simulink model "k6jca_181222_SHERA_2_subsample"  (R2018b)
settings: Solver=ode45  StartTime=0.0  StopTime=10000  MaxStep=1  RelTol=1e-3  EnableMultiTasking=on
InitFcn:
  | D=30
settings Model: Creator=Dick  LastModifiedBy=Jeff
settings DataIOCC: LimitDataPoints=on  SaveFormat=Array  SaveOutput=off  SignalLogging=off  DSMLogging=off  SaveTime=off
settings OptimizationCC: LifeSpan=inf
settings DebuggingCC: SFUnexpectedBacktrackingDiag=warning  SFNoUnconditionalDefaultTransitionDiag=warning  SFExecutionAtInitializationDiag=none
settings HardwareCC: ProdBitPerPointer=32  ProdBitPerSizeT=32  ProdBitPerPtrDiffT=32  ProdLargestAtomicFloat=None  ProdIntDivRoundTo=Undefined  ProdEndianess=Unspecified  ProdWordSize=32  ProdHWDeviceType=32-bit Generic
settings ModelReferenceCC: PropagateSignalLabelsOutOfModel=off
settings SFSimCC: SimUseLocalCustomCode=off
settings RTWCC: RTWUseLocalCustomCode=off
settings CodeAppCC: StateflowObjectComments=on
settings GRTTargetCC: TargetLangStandard=C89/C90 (ANSI)  GeneratePreprocessorConditionals=Disable all
settings ConfigComp: CovMetricSettings=dw  CovHtmlReporting=on  CovSaveCumulativeToWorkspaceVar=on  CovSaveSingleToWorkspaceVar=on  CovExternalEMLEnable=off

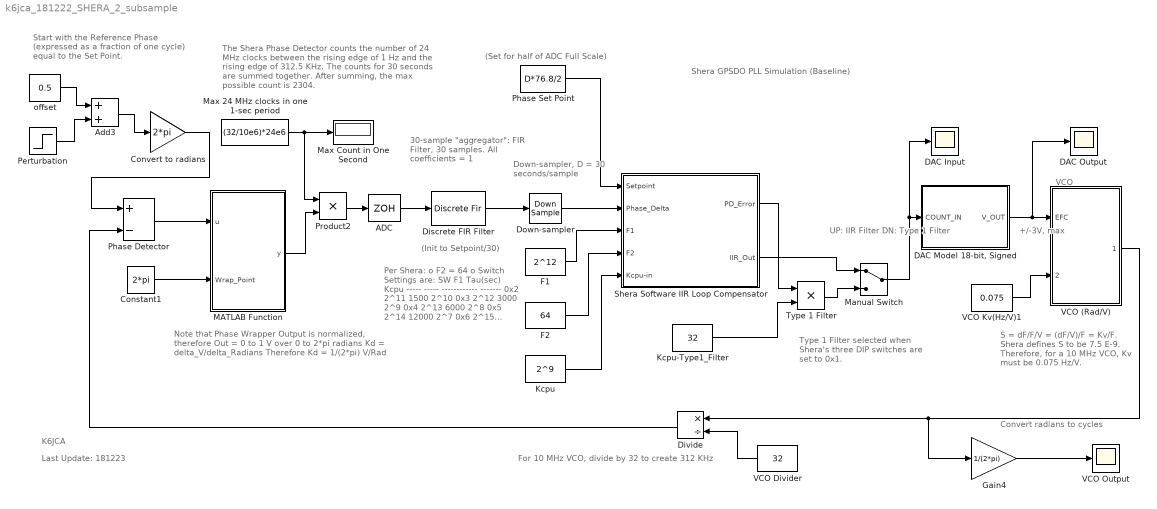
== system k6jca_181222_SHERA_2_subsample ==
  note: Down-sampler,
      | D = 30
      | seconds/sample
  note: Last Update: 181223
  note: (Set for half of ADC Full Scale)
  note: 30-sample "aggregator":
      | FIR Filter,
      | 30 samples.
      | All coefficients = 1
  note: Start with the Reference Phase
      | (expressed as a fraction of one cycle)
      | equal to the Set Point.
  note: UP:  IIR Filter
      | DN:  Type 1 Filter
  note: Type 1 Filter selected
      | when Shera's three
      | DIP switches are set to 0x1.
  note: S = dF/F/V = (dF/V)/F = Kv/F.
      | Shera defines S to be 7.5 E-9.
      | Therefore, for a 10 MHz VCO,
      | Kv must be 0.075 Hz/V.
  note: The Shera Phase Detector counts the number of 24 MHz clocks between the rising edge of 1 Hz and the rising edge of 312.5 KHz.
      |
      | The counts for 30 seconds are summed together.  After summing,  the max possible count is 2304.
  note: Per Shera:
      |      o  F2 = 64
      |      o  Switch Settings are:
      |
      |    SW      F1     Tau(sec)    Kcpu
      |    -----     -----    ------------   -------
      |    0x2     2^11      1500       2^10
      |    0x3     2^12      3000       2^9
      |    0x4     2^13      6000       2^8
      |    0x5     2^14    12000       2^7
      |    0x6     2^15    24000       2^6
      |    0x7     2^16    48000       2^5
  note: For 10 MHz VCO, divide by 32 to create 312 KHz
  note: +/-3V,
      |  max
  note: K6JCA
  note: Shera GPSDO PLL Simulation
      | (Baseline)
  note: Convert radians to cycles
  note: Note that Phase Wrapper Output is normalized,
      | therefore Out =  0 to 1 V over 0 to 2*pi radians
      |
      | Kd = delta_V/delta_Radians
      | Therefore Kd = 1/(2*pi)  V/Rad
  note: VCO
  note: (Init to Setpoint/30)
  ADC : ZeroOrderHold
  Add3 : Sum
  Constant1 : Constant  Value=2*pi  SampleTime=Inf
  "Convert to radians " : Gain  Gain=2*pi
  DAC Input : Scope
  "DAC Model 18-bit, Signed" : Subsystem
  DAC Output : Scope
  Discrete FIR Filter : DiscreteFir  Coefficients=[1 1 1 1 1 1 1 1 1 1 1 1 1 1 1 1 1 1 1 1 1 1 1 1 1 1 1 1 1 1]  InitialStates=76.8/2
  Divide : Product  Inputs=*/
  "Down-sampler " : DownSample  N=D  RateOptions=Allow multirate processing
  F1 : Constant  Value=2^12  SampleTime=Inf
  F2 : Constant  Value=64  SampleTime=Inf
  Gain4 : Gain  Gain=1/(2*pi)
  Kcpu : Constant  Value=2^9  SampleTime=Inf
  Kcpu-Type1_Filter : Constant  Value=32  SampleTime=Inf
  MATLAB Function : MATLAB Function  TreatAsAtomicUnit=on
  Manual Switch : ManualSwitch
  Max 24 MHz clocks in one 1-sec period : Constant  Value=(32/10e6)*24e6  SampleTime=Inf
  Max Count in One Second : Display
  "Perturbation " : Step  Time=100  After=0.49  SampleTime=1
  Phase Detector : Sum  Inputs=+-
  Phase Set Point : Constant  Value=D*76.8/2  SampleTime=Inf
  Product2 : Product
  "Shera Software IIR Loop Compensator " : Subsystem
  Type 1 Filter : Product  Inputs=**
  VCO (Rad/V) : Subsystem
  VCO Divider : Constant  Value=32  SampleTime=Inf
  VCO Kv(Hz/V)1 : Constant  Value=0.075  SampleTime=Inf
  VCO Output : Scope
  offset : Constant  Value=0.5  SampleTime=Inf
  wires:
  "Perturbation "/1 -> Add3/2
  Phase Detector/1 -> MATLAB Function/1(u)
  Constant1/1 -> MATLAB Function/2(Wrap_Point)
  Product2/1 -> ADC/1
  "Convert to radians "/1 -> Phase Detector/1
  "Shera Software IIR Loop Compensator "/1("PD_Error ") -> Type 1 Filter/1
  VCO (Rad/V)/1(Radians) -> Divide/1, Gain4/1
  F2/1 -> "Shera Software IIR Loop Compensator "/4(F2)
  F1/1 -> "Shera Software IIR Loop Compensator "/3(F1)
  Kcpu/1 -> "Shera Software IIR Loop Compensator "/5(Kcpu-in)
  VCO Kv(Hz/V)1/1 -> VCO (Rad/V)/2(Kv_(Hz/V))
  "DAC Model 18-bit, Signed"/1(V_OUT) -> DAC Output/1, VCO (Rad/V)/1(EFC)
  VCO Divider/1 -> Divide/2
  Manual Switch/1 -> DAC Input/1, "DAC Model 18-bit, Signed"/1(COUNT_IN)
  Kcpu-Type1_Filter/1 -> Type 1 Filter/2
  Type 1 Filter/1 -> Manual Switch/2
  "Shera Software IIR Loop Compensator "/2("IIR_Out ") -> Manual Switch/1
  Phase Set Point/1 -> "Shera Software IIR Loop Compensator "/1(Setpoint)
  "Down-sampler "/1 -> "Shera Software IIR Loop Compensator "/2(Phase_Delta)
  Discrete FIR Filter/1 -> "Down-sampler "/1
  ADC/1 -> Discrete FIR Filter/1
  offset/1 -> Add3/1
  Divide/1 -> Phase Detector/2
  MATLAB Function/1(y) -> Product2/2
  Max 24 MHz clocks in one 1-sec period/1 -> Max Count in One Second/1, Product2/1
  Add3/1 -> "Convert to radians "/1
  Gain4/1 -> VCO Output/1

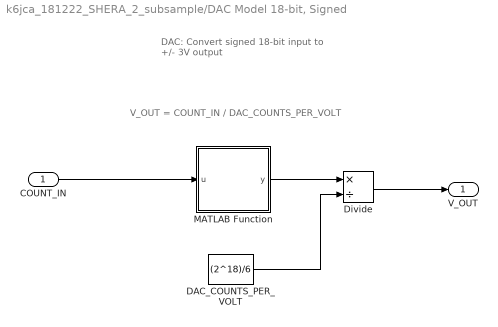
== system k6jca_181222_SHERA_2_subsample/DAC Model 18-bit, Signed ==
  note: V_OUT = COUNT_IN / DAC_COUNTS_PER_VOLT
  note: DAC:
      | Convert signed 18-bit input
      | to
      | +/- 3V output
  COUNT_IN : Inport
  "DAC_COUNTS_PER_VOLT " : Constant  Value=(2^18)/6  SampleTime=Inf
  Divide : Product  Inputs=*/
  MATLAB Function : MATLAB Function  TreatAsAtomicUnit=on
  V_OUT : Outport
  wires:
  "DAC_COUNTS_PER_VOLT "/1 -> Divide/2
  Divide/1 -> V_OUT/1
  MATLAB Function/1(y) -> Divide/1
  COUNT_IN/1 -> MATLAB Function/1(u)

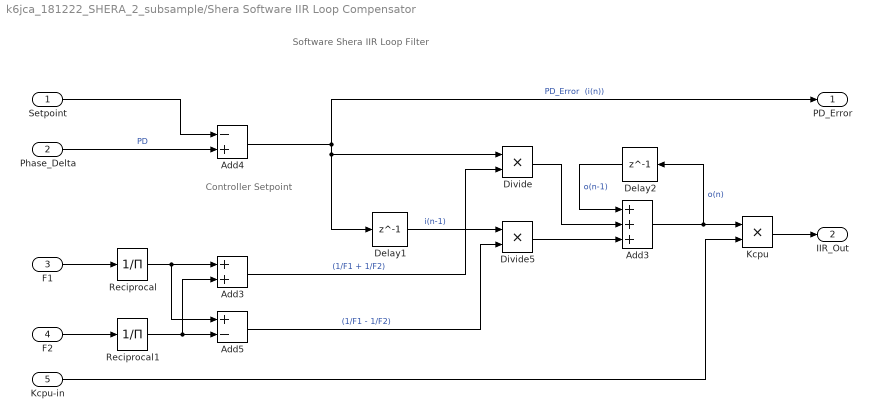
== system k6jca_181222_SHERA_2_subsample/Shera Software IIR Loop Compensator  ==
  note: Software Shera IIR Loop Filter
  note: Controller
      | Setpoint
  Setpoint : Inport
  Phase_Delta : Inport  Port=2
  F1 : Inport  Port=3
  F2 : Inport  Port=4
  Kcpu-in : Inport  Port=5
  Add3 : Sum
  "Add3 " : Sum  Inputs=+++
  Add4 : Sum  Inputs=-+
  Add5 : Sum  Inputs=+-
  Delay1 : Delay  DelayLength=1
  Delay2 : Delay  DelayLength=1
  Divide : Product  Inputs=**
  Divide5 : Product  Inputs=**
  Kcpu : Product  Inputs=**
  Reciprocal : Product  Inputs=/
  Reciprocal1 : Product  Inputs=/
  "PD_Error " : Outport
  "IIR_Out " : Outport  Port=2
  wires:
  Setpoint/1 -> Add4/1
  Add4/1 -> Divide/1, Delay1/1, "PD_Error "/1  "PD_Error  (i(n))"
  "Add3 "/1 -> Delay2/1, Kcpu/1  "o(n)"
  F1/1 -> Reciprocal/1
  F2/1 -> Reciprocal1/1
  Reciprocal/1 -> Add5/1, Add3/1
  Reciprocal1/1 -> Add5/2, Add3/2
  Add3/1 -> Divide/2  "(1/F1 + 1/F2)"
  Delay1/1 -> Divide5/1  "i(n-1)"
  Add5/1 -> Divide5/2  "(1/F1 - 1/F2)"
  Delay2/1 -> "Add3 "/1  "o(n-1)"
  Divide/1 -> "Add3 "/2
  Divide5/1 -> "Add3 "/3
  Phase_Delta/1 -> Add4/2  "PD"
  Kcpu-in/1 -> Kcpu/2
  Kcpu/1 -> "IIR_Out "/1

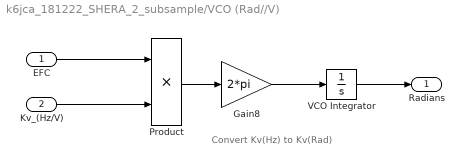
== system k6jca_181222_SHERA_2_subsample/VCO (Rad//V) ==
  note: Convert Kv(Hz)
      | to Kv(Rad)
  EFC : Inport
  Kv_(Hz/V) : Inport  Port=2
  Gain8 : Gain  Gain=2*pi
  Product : Product
  VCO Integrator : Integrator
  Radians : Outport
  wires:
  Gain8/1 -> VCO Integrator/1
  EFC/1 -> Product/1
  Product/1 -> Gain8/1
  VCO Integrator/1 -> Radians/1
  Kv_(Hz/V)/1 -> Product/2

== matlab function k6jca_181222_SHERA_2_subsample/MATLAB Function ==
  data: u input; y output; Wrap_Point input
function y = phase_wrapper(u,Wrap_Point)
%#codegen
y=0;
if u > 0
   y = mod(u,Wrap_Point);
elseif u < 0
   y = Wrap_Point-(mod(-u,Wrap_Point));  
end
y = y/Wrap_Point;  % normalize y to 1.

== matlab function k6jca_181222_SHERA_2_subsample/DAC Model 18-bit, Signed/MATLAB Function ==
  data: u input; y output
function y = dac_limiter(u)
%#codegen
% This limits the DAC input to +131071
% and to -131072 (18 bit range).

y = u;
if u > 131071
   y = 131071;
elseif u < -131072
   y = -131072;  
end
